simulink model "HybridFEMModel"  (Simulink 7.0)
settings: Solver=FixedStepDiscrete  SolverMode=SingleTasking  StartTime=0.0  StopTime=RunningTime  FixedStep=SampleRate  RelTol=1e-3
values from neighbouring files (symbols this model uses):
  SampleRate = Integrator.Timestep    [HybridFEMSetup_2.m]
undefined symbols (not defined in the file or in its folder): Elements
libraries: simulink x2
(part 1 of 3)
settings Model: Creator=Tommy  LastModifiedBy=Tommy

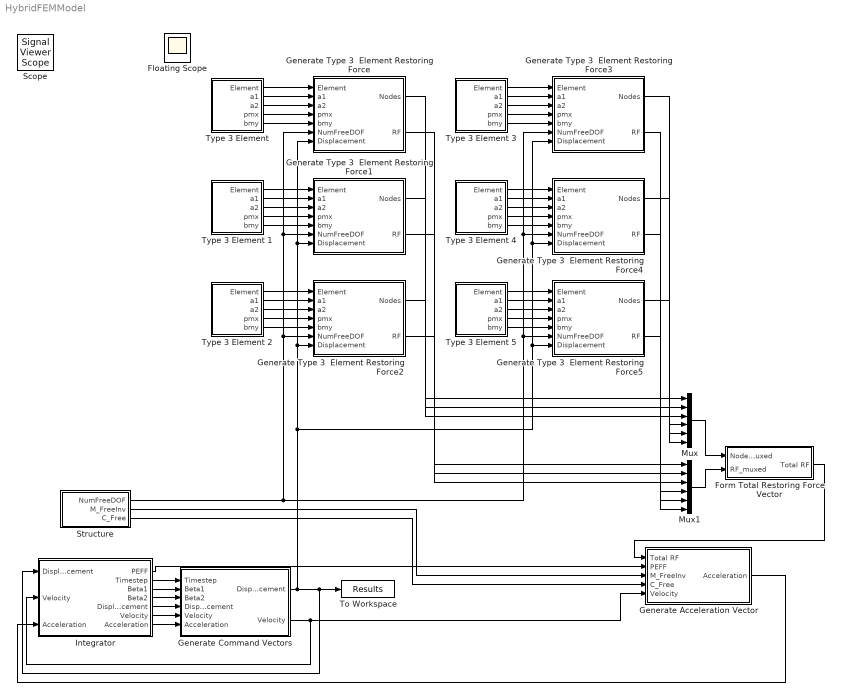
== system HybridFEMModel ==
  Form Total Restoring Force Vector : Subsystem
      mask Type: Form Restoring Force Vector
      mask Description:
      | Takes the restoring force vectors from each Element and combines them to form a total restoring force vector.
      | 
      | Connect the "Nodes_muxed" signal to the output of a Mux block which takes in all the Element "Nodes" outputs in order of ID.
      | 
      | Connect the "RF_muxed" signal to the output of a Mux block which takes in all the Element "RF" outputs in order of ID.
  Generate Acceleration Vector : Subsystem
      mask Type: Generate Acceleration Vector
      mask Description:
      | Takes the total restoring force vector and Integration parameters and generates the next step acceleration vector.
      | 
      | Connect the "Total RF" input to the output of the "Form Total Restoring Force Vector" block.
      | 
      | Connect the "PEFF", "M_Free_Inv" (MassMatrixFreeInv) and "C_Free" (DampingMatrixFree) to the "Structure" block.
      | 
      | Connect the "Velocity" input to the output of the "Generate Command Vectors" block
  Generate Command Vectors : Subsystem
      mask Type: Generate Command Vectors
      mask Description:
      | Generates the Displacement and Velocity vectors using the CR Algorithm.
      | 
      | Connect all inputs to the outputs of the "Integrator" block.
  Generate Type 3  Element Restoring Force : Subsystem
      mask Type: Generate Type 3 Element Restoring Force
      mask Description:
      | Generates the Restoring Force vector for a Type 3 Element
      | 
      | Connect the "Element" input to a "Type 3 Element" block.
      | 
      | Connect the "a1", "a2", "pmx" and "bmy" inputs to the outputs of the "Type 3 Element" block.
      | 
      | Connect the "NumFreeDOF" input to the output of a "Structure" block.
      | 
      | Connect the "Displacement" input to the output of the "Generate Command Vectors" block.
  Generate Type 3  Element Restoring Force1 : Subsystem
      mask Type: Generate Type 3 Element Restoring Force
      mask Description:
      | Generates the Restoring Force vector for a Type 3 Element
      | 
      | Connect the "Element" input to a "Type 3 Element" block.
      | 
      | Connect the "a1", "a2", "pmx" and "bmy" inputs to the outputs of the "Type 3 Element" block.
      | 
      | Connect the "NumFreeDOF" input to the output of a "Structure" block.
      | 
      | Connect the "Displacement" input to the output of the "Generate Command Vectors" block.
  Generate Type 3  Element Restoring Force2 : Subsystem
      mask Type: Generate Type 3 Element Restoring Force
      mask Description:
      | Generates the Restoring Force vector for a Type 3 Element
      | 
      | Connect the "Element" input to a "Type 3 Element" block.
      | 
      | Connect the "a1", "a2", "pmx" and "bmy" inputs to the outputs of the "Type 3 Element" block.
      | 
      | Connect the "NumFreeDOF" input to the output of a "Structure" block.
      | 
      | Connect the "Displacement" input to the output of the "Generate Command Vectors" block.
  Generate Type 3  Element Restoring Force3 : Subsystem
      mask Type: Generate Type 3 Element Restoring Force
      mask Description:
      | Generates the Restoring Force vector for a Type 3 Element
      | 
      | Connect the "Element" input to a "Type 3 Element" block.
      | 
      | Connect the "a1", "a2", "pmx" and "bmy" inputs to the outputs of the "Type 3 Element" block.
      | 
      | Connect the "NumFreeDOF" input to the output of a "Structure" block.
      | 
      | Connect the "Displacement" input to the output of the "Generate Command Vectors" block.
  Generate Type 3  Element Restoring Force4 : Subsystem
      mask Type: Generate Type 3 Element Restoring Force
      mask Description:
      | Generates the Restoring Force vector for a Type 3 Element
      | 
      | Connect the "Element" input to a "Type 3 Element" block.
      | 
      | Connect the "a1", "a2", "pmx" and "bmy" inputs to the outputs of the "Type 3 Element" block.
      | 
      | Connect the "NumFreeDOF" input to the output of a "Structure" block.
      | 
      | Connect the "Displacement" input to the output of the "Generate Command Vectors" block.
  Generate Type 3  Element Restoring Force5 : Subsystem
      mask Type: Generate Type 3 Element Restoring Force
      mask Description:
      | Generates the Restoring Force vector for a Type 3 Element
      | 
      | Connect the "Element" input to a "Type 3 Element" block.
      | 
      | Connect the "a1", "a2", "pmx" and "bmy" inputs to the outputs of the "Type 3 Element" block.
      | 
      | Connect the "NumFreeDOF" input to the output of a "Structure" block.
      | 
      | Connect the "Displacement" input to the output of the "Generate Command Vectors" block.
  Integrator : Subsystem
      mask Type: Integrator
      mask Description:
      | The Integrator structure is pulled from the MATLAB workspace after running the initialization script.
      | 
      | Connect the Displacement and Velocity inputs to the outputs of the "Generate Command Vectors" block.
      | 
      | Connect the Acceleration input to the output of the "Generate Acceleration Vector" block
  Mux : Mux  Inputs=6
  Mux1 : Mux  Inputs=6
  Structure : Subsystem
      mask Type: Structure Data Source
      mask Description: The Structure data is pulled from the MATLAB workspace after running the initialization file
  To Workspace : ToWorkspace  VariableName=Results  SampleTime=SampleRate  SaveFormat=Array
  "Type 3 Element " : Subsystem  mask(Element Type 3){id=1}
      mask prompts: id "Element ID:"
      mask help: Enter the ID for this element corresponding with the input configuration file
  Type 3 Element 1 : Subsystem  mask(Element Type 3){id=2}
      mask prompts: id "Element ID:"
      mask help: Enter the ID for this element corresponding with the input configuration file
  Type 3 Element 2 : Subsystem  mask(Element Type 3){id=3}
      mask prompts: id "Element ID:"
      mask help: Enter the ID for this element corresponding with the input configuration file
  Type 3 Element 3 : Subsystem  mask(Element Type 3){id=4}
      mask prompts: id "Element ID:"
      mask help: Enter the ID for this element corresponding with the input configuration file
  Type 3 Element 4 : Subsystem  mask(Element Type 3){id=5}
      mask prompts: id "Element ID:"
      mask help: Enter the ID for this element corresponding with the input configuration file
  Type 3 Element 5 : Subsystem  mask(Element Type 3){id=6}
      mask prompts: id "Element ID:"
      mask help: Enter the ID for this element corresponding with the input configuration file
  Floating Scope : Scope
      settings: Floating=on
  Scope : SignalViewerScope  IOType=viewer  RefreshTime=0.035000
  wires:
  Integrator/5(Displacement) -> Generate Command Vectors/4("Displacement ")
  Generate Command Vectors/1(Displacement) -> Integrator/1("Displacement "), To Workspace/1, Generate Type 3  Element Restoring Force2/7(Displacement), Generate Type 3  Element Restoring Force1/7(Displacement), Generate Type 3  Element Restoring Force/7(Displacement), Generate Type 3  Element Restoring Force5/7(Displacement), Generate Type 3  Element Restoring Force4/7(Displacement), Generate Type 3  Element Restoring Force3/7(Displacement)
  Form Total Restoring Force Vector/1(Total RF) -> Generate Acceleration Vector/1(Total RF)
  Mux/1 -> Form Total Restoring Force Vector/1(Nodes_Muxed)
  Mux1/1 -> Form Total Restoring Force Vector/2(RF_muxed)
  Integrator/1(PEFF) -> Generate Acceleration Vector/2(PEFF)
  Generate Command Vectors/2(Velocity) -> Integrator/2("Velocity "), Generate Acceleration Vector/5(Velocity)
  Structure/2(M_FreeInv) -> Generate Acceleration Vector/3(M_FreeInv)
  Structure/3(C_Free) -> Generate Acceleration Vector/4(C_Free)
  Generate Acceleration Vector/1(Acceleration) -> Integrator/3("Acceleration ")
  Integrator/2(Timestep) -> Generate Command Vectors/1(Timestep)
  Integrator/3(Beta1) -> Generate Command Vectors/2(Beta1)
  Integrator/4(Beta2) -> Generate Command Vectors/3(Beta2)
  Integrator/6(Velocity) -> Generate Command Vectors/5("Velocity ")
  Integrator/7(Acceleration) -> Generate Command Vectors/6(Acceleration)
  "Type 3 Element "/1(Element) -> Generate Type 3  Element Restoring Force/1(Element)
  "Type 3 Element "/2(a1) -> Generate Type 3  Element Restoring Force/2(a1)
  "Type 3 Element "/3(a2) -> Generate Type 3  Element Restoring Force/3(a2)
  "Type 3 Element "/4(pmx) -> Generate Type 3  Element Restoring Force/4(pmx)
  Type 3 Element 1/1(Element) -> Generate Type 3  Element Restoring Force1/1(Element)
  Type 3 Element 1/2(a1) -> Generate Type 3  Element Restoring Force1/2(a1)
  Type 3 Element 1/3(a2) -> Generate Type 3  Element Restoring Force1/3(a2)
  Type 3 Element 1/4(pmx) -> Generate Type 3  Element Restoring Force1/4(pmx)
  Type 3 Element 1/5(bmy) -> Generate Type 3  Element Restoring Force1/5(bmy)
  Type 3 Element 2/1(Element) -> Generate Type 3  Element Restoring Force2/1(Element)
  Type 3 Element 2/2(a1) -> Generate Type 3  Element Restoring Force2/2(a1)
  Type 3 Element 2/3(a2) -> Generate Type 3  Element Restoring Force2/3(a2)
  Type 3 Element 2/4(pmx) -> Generate Type 3  Element Restoring Force2/4(pmx)
  Type 3 Element 2/5(bmy) -> Generate Type 3  Element Restoring Force2/5(bmy)
  Type 3 Element 3/1(Element) -> Generate Type 3  Element Restoring Force3/1(Element)
  Type 3 Element 3/2(a1) -> Generate Type 3  Element Restoring Force3/2(a1)
  Type 3 Element 3/3(a2) -> Generate Type 3  Element Restoring Force3/3(a2)
  Type 3 Element 3/4(pmx) -> Generate Type 3  Element Restoring Force3/4(pmx)
  Type 3 Element 3/5(bmy) -> Generate Type 3  Element Restoring Force3/5(bmy)
  Type 3 Element 4/1(Element) -> Generate Type 3  Element Restoring Force4/1(Element)
  Type 3 Element 4/2(a1) -> Generate Type 3  Element Restoring Force4/2(a1)
  Type 3 Element 4/3(a2) -> Generate Type 3  Element Restoring Force4/3(a2)
  Type 3 Element 4/4(pmx) -> Generate Type 3  Element Restoring Force4/4(pmx)
  Type 3 Element 4/5(bmy) -> Generate Type 3  Element Restoring Force4/5(bmy)
  Type 3 Element 5/1(Element) -> Generate Type 3  Element Restoring Force5/1(Element)
  Type 3 Element 5/2(a1) -> Generate Type 3  Element Restoring Force5/2(a1)
  Type 3 Element 5/3(a2) -> Generate Type 3  Element Restoring Force5/3(a2)
  Type 3 Element 5/4(pmx) -> Generate Type 3  Element Restoring Force5/4(pmx)
  Type 3 Element 5/5(bmy) -> Generate Type 3  Element Restoring Force5/5(bmy)
  "Type 3 Element "/5(bmy) -> Generate Type 3  Element Restoring Force/5(bmy)
  Structure/1(NumFreeDOF) -> Generate Type 3  Element Restoring Force/6(NumFreeDOF), Generate Type 3  Element Restoring Force1/6(NumFreeDOF), Generate Type 3  Element Restoring Force2/6(NumFreeDOF), Generate Type 3  Element Restoring Force3/6(NumFreeDOF), Generate Type 3  Element Restoring Force4/6(NumFreeDOF), Generate Type 3  Element Restoring Force5/6(NumFreeDOF)
  Generate Type 3  Element Restoring Force/1(Nodes) -> Mux/1
  Generate Type 3  Element Restoring Force1/1(Nodes) -> Mux/2
  Generate Type 3  Element Restoring Force2/1(Nodes) -> Mux/3
  Generate Type 3  Element Restoring Force3/1(Nodes) -> Mux/4
  Generate Type 3  Element Restoring Force4/1(Nodes) -> Mux/5
  Generate Type 3  Element Restoring Force5/1(Nodes) -> Mux/6
  Generate Type 3  Element Restoring Force/2(RF) -> Mux1/1
  Generate Type 3  Element Restoring Force1/2(RF) -> Mux1/2
  Generate Type 3  Element Restoring Force2/2(RF) -> Mux1/3
  Generate Type 3  Element Restoring Force3/2(RF) -> Mux1/4
  Generate Type 3  Element Restoring Force4/2(RF) -> Mux1/5
  Generate Type 3  Element Restoring Force5/2(RF) -> Mux1/6

== system HybridFEMModel/Form Total Restoring Force Vector ==
  Nodes_Muxed : Inport  OutDataType=sfix(16)  OutScaling=2^0
  RF_muxed : Inport  Port=2  OutDataType=sfix(16)  OutScaling=2^0
  Form Restoring Force Vector : Stateflow chart
  Total RF : Outport  OutDataType=sfix(16)  OutScaling=2^0
  wires:
  RF_muxed/1 -> Form Restoring Force Vector/2(RF_muxed)
  Form Restoring Force Vector/1(TotalRF) -> Total RF/1
  Nodes_Muxed/1 -> Form Restoring Force Vector/1(Nodes_muxed)

== system HybridFEMModel/Generate Acceleration Vector ==
  Total RF : Inport  OutDataType=sfix(16)  OutScaling=2^0
  PEFF : Inport  Port=2  OutDataType=sfix(16)  OutScaling=2^0
  M_FreeInv : Inport  Port=3  OutDataType=sfix(16)  OutScaling=2^0
  C_Free : Inport  Port=4  OutDataType=sfix(16)  OutScaling=2^0
  Velocity : Inport  Port=5  OutDataType=sfix(16)  OutScaling=2^0
  Generate Acceleration Vector : Stateflow chart
  Step Count : Subsystem
      mask Type: Step count
      mask Description: Generates the step count
  Acceleration : Outport  OutDataType=sfix(16)  OutScaling=2^0
  wires:
  Step Count/1(Step Count) -> Generate Acceleration Vector/6(step_count)
  Total RF/1 -> Generate Acceleration Vector/1(TotalRF)
  Generate Acceleration Vector/1(Acceleration) -> Acceleration/1
  PEFF/1 -> Generate Acceleration Vector/2(PEFF)
  M_FreeInv/1 -> Generate Acceleration Vector/3(M_FreeInv)
  C_Free/1 -> Generate Acceleration Vector/4(C_Free)
  Velocity/1 -> Generate Acceleration Vector/5(Velocity)

== system HybridFEMModel/Generate Command Vectors ==
  Timestep : Inport  OutDataType=sfix(16)  OutScaling=2^0
  Beta1 : Inport  Port=2  OutDataType=sfix(16)  OutScaling=2^0
  Beta2 : Inport  Port=3  OutDataType=sfix(16)  OutScaling=2^0
  "Displacement " : Inport  Port=4  OutDataType=sfix(16)  OutScaling=2^0
  "Velocity " : Inport  Port=5  OutDataType=sfix(16)  OutScaling=2^0
  Acceleration : Inport  Port=6  OutDataType=sfix(16)  OutScaling=2^0
  Generate Command Vectors : Stateflow chart
  Displacement : Outport  OutDataType=sfix(16)  OutScaling=2^0
  Velocity : Outport  Port=2  OutDataType=sfix(16)  OutScaling=2^0
  wires:
  Generate Command Vectors/1(Displacement_v) -> Displacement/1
  Generate Command Vectors/2(Velocity_v) -> Velocity/1
  Timestep/1 -> Generate Command Vectors/1(Timestep)
  Beta1/1 -> Generate Command Vectors/2(Beta1)
  Beta2/1 -> Generate Command Vectors/3(Beta2)
  "Displacement "/1 -> Generate Command Vectors/4(Displacement)
  "Velocity "/1 -> Generate Command Vectors/5(Velocity)
  Acceleration/1 -> Generate Command Vectors/6(Acceleration)

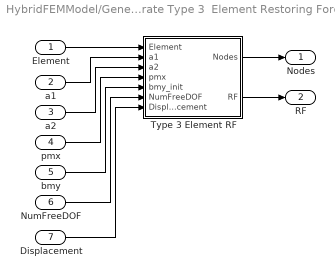
== system HybridFEMModel/Generate Type 3  Element Restoring Force ==
  Element : Inport  OutDataType=sfix(16)  OutScaling=2^0
  a1 : Inport  Port=2  OutDataType=sfix(16)  OutScaling=2^0
  a2 : Inport  Port=3  OutDataType=sfix(16)  OutScaling=2^0
  pmx : Inport  Port=4  OutDataType=sfix(16)  OutScaling=2^0
  bmy : Inport  Port=5  OutDataType=sfix(16)  OutScaling=2^0
  NumFreeDOF : Inport  Port=6  OutDataType=sfix(16)  OutScaling=2^0
  Displacement : Inport  Port=7  OutDataType=sfix(16)  OutScaling=2^0
  Type 3 Element RF : Stateflow chart
  Nodes : Outport  OutDataType=sfix(16)  OutScaling=2^0
  RF : Outport  Port=2  OutDataType=sfix(16)  OutScaling=2^0
  wires:
  Type 3 Element RF/1(Nodes) -> Nodes/1
  Type 3 Element RF/2(RF) -> RF/1
  Element/1 -> Type 3 Element RF/1(Element)
  a1/1 -> Type 3 Element RF/2(a1)
  a2/1 -> Type 3 Element RF/3(a2)
  pmx/1 -> Type 3 Element RF/4(pmx)
  bmy/1 -> Type 3 Element RF/5(bmy_init)
  NumFreeDOF/1 -> Type 3 Element RF/6(NumFreeDOF)
  Displacement/1 -> Type 3 Element RF/7(Displacement)

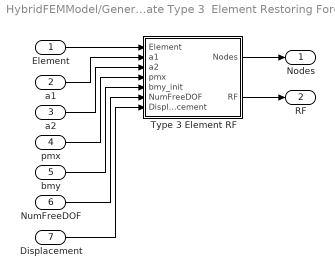
== system HybridFEMModel/Generate Type 3  Element Restoring Force1 ==
  Element : Inport  OutDataType=sfix(16)  OutScaling=2^0
  a1 : Inport  Port=2  OutDataType=sfix(16)  OutScaling=2^0
  a2 : Inport  Port=3  OutDataType=sfix(16)  OutScaling=2^0
  pmx : Inport  Port=4  OutDataType=sfix(16)  OutScaling=2^0
  bmy : Inport  Port=5  OutDataType=sfix(16)  OutScaling=2^0
  NumFreeDOF : Inport  Port=6  OutDataType=sfix(16)  OutScaling=2^0
  Displacement : Inport  Port=7  OutDataType=sfix(16)  OutScaling=2^0
  Type 3 Element RF : Stateflow chart
  Nodes : Outport  OutDataType=sfix(16)  OutScaling=2^0
  RF : Outport  Port=2  OutDataType=sfix(16)  OutScaling=2^0
  wires:
  Displacement/1 -> Type 3 Element RF/7(Displacement)
  NumFreeDOF/1 -> Type 3 Element RF/6(NumFreeDOF)
  bmy/1 -> Type 3 Element RF/5(bmy_init)
  pmx/1 -> Type 3 Element RF/4(pmx)
  a2/1 -> Type 3 Element RF/3(a2)
  a1/1 -> Type 3 Element RF/2(a1)
  Element/1 -> Type 3 Element RF/1(Element)
  Type 3 Element RF/2(RF) -> RF/1
  Type 3 Element RF/1(Nodes) -> Nodes/1

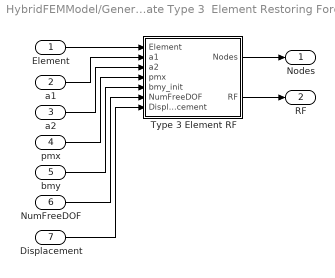
== system HybridFEMModel/Generate Type 3  Element Restoring Force2 ==
  Element : Inport  OutDataType=sfix(16)  OutScaling=2^0
  a1 : Inport  Port=2  OutDataType=sfix(16)  OutScaling=2^0
  a2 : Inport  Port=3  OutDataType=sfix(16)  OutScaling=2^0
  pmx : Inport  Port=4  OutDataType=sfix(16)  OutScaling=2^0
  bmy : Inport  Port=5  OutDataType=sfix(16)  OutScaling=2^0
  NumFreeDOF : Inport  Port=6  OutDataType=sfix(16)  OutScaling=2^0
  Displacement : Inport  Port=7  OutDataType=sfix(16)  OutScaling=2^0
  Type 3 Element RF : Stateflow chart
  Nodes : Outport  OutDataType=sfix(16)  OutScaling=2^0
  RF : Outport  Port=2  OutDataType=sfix(16)  OutScaling=2^0
  wires:
  Type 3 Element RF/1(Nodes) -> Nodes/1
  Type 3 Element RF/2(RF) -> RF/1
  Element/1 -> Type 3 Element RF/1(Element)
  a1/1 -> Type 3 Element RF/2(a1)
  a2/1 -> Type 3 Element RF/3(a2)
  pmx/1 -> Type 3 Element RF/4(pmx)
  bmy/1 -> Type 3 Element RF/5(bmy_init)
  NumFreeDOF/1 -> Type 3 Element RF/6(NumFreeDOF)
  Displacement/1 -> Type 3 Element RF/7(Displacement)

== system HybridFEMModel/Generate Type 3  Element Restoring Force3 ==
  Element : Inport  OutDataType=sfix(16)  OutScaling=2^0
  a1 : Inport  Port=2  OutDataType=sfix(16)  OutScaling=2^0
  a2 : Inport  Port=3  OutDataType=sfix(16)  OutScaling=2^0
  pmx : Inport  Port=4  OutDataType=sfix(16)  OutScaling=2^0
  bmy : Inport  Port=5  OutDataType=sfix(16)  OutScaling=2^0
  NumFreeDOF : Inport  Port=6  OutDataType=sfix(16)  OutScaling=2^0
  Displacement : Inport  Port=7  OutDataType=sfix(16)  OutScaling=2^0
  Type 3 Element RF : Stateflow chart
  Nodes : Outport  OutDataType=sfix(16)  OutScaling=2^0
  RF : Outport  Port=2  OutDataType=sfix(16)  OutScaling=2^0
  wires:
  Displacement/1 -> Type 3 Element RF/7(Displacement)
  NumFreeDOF/1 -> Type 3 Element RF/6(NumFreeDOF)
  bmy/1 -> Type 3 Element RF/5(bmy_init)
  pmx/1 -> Type 3 Element RF/4(pmx)
  a2/1 -> Type 3 Element RF/3(a2)
  a1/1 -> Type 3 Element RF/2(a1)
  Element/1 -> Type 3 Element RF/1(Element)
  Type 3 Element RF/2(RF) -> RF/1
  Type 3 Element RF/1(Nodes) -> Nodes/1

== system HybridFEMModel/Generate Type 3  Element Restoring Force4 ==
  Element : Inport  OutDataType=sfix(16)  OutScaling=2^0
  a1 : Inport  Port=2  OutDataType=sfix(16)  OutScaling=2^0
  a2 : Inport  Port=3  OutDataType=sfix(16)  OutScaling=2^0
  pmx : Inport  Port=4  OutDataType=sfix(16)  OutScaling=2^0
  bmy : Inport  Port=5  OutDataType=sfix(16)  OutScaling=2^0
  NumFreeDOF : Inport  Port=6  OutDataType=sfix(16)  OutScaling=2^0
  Displacement : Inport  Port=7  OutDataType=sfix(16)  OutScaling=2^0
  Type 3 Element RF : Stateflow chart
  Nodes : Outport  OutDataType=sfix(16)  OutScaling=2^0
  RF : Outport  Port=2  OutDataType=sfix(16)  OutScaling=2^0
  wires:
  Type 3 Element RF/1(Nodes) -> Nodes/1
  Type 3 Element RF/2(RF) -> RF/1
  Element/1 -> Type 3 Element RF/1(Element)
  a1/1 -> Type 3 Element RF/2(a1)
  a2/1 -> Type 3 Element RF/3(a2)
  pmx/1 -> Type 3 Element RF/4(pmx)
  bmy/1 -> Type 3 Element RF/5(bmy_init)
  NumFreeDOF/1 -> Type 3 Element RF/6(NumFreeDOF)
  Displacement/1 -> Type 3 Element RF/7(Displacement)

== system HybridFEMModel/Generate Type 3  Element Restoring Force5 ==
  Element : Inport  OutDataType=sfix(16)  OutScaling=2^0
  a1 : Inport  Port=2  OutDataType=sfix(16)  OutScaling=2^0
  a2 : Inport  Port=3  OutDataType=sfix(16)  OutScaling=2^0
  pmx : Inport  Port=4  OutDataType=sfix(16)  OutScaling=2^0
  bmy : Inport  Port=5  OutDataType=sfix(16)  OutScaling=2^0
  NumFreeDOF : Inport  Port=6  OutDataType=sfix(16)  OutScaling=2^0
  Displacement : Inport  Port=7  OutDataType=sfix(16)  OutScaling=2^0
  Type 3 Element RF : Stateflow chart
  Nodes : Outport  OutDataType=sfix(16)  OutScaling=2^0
  RF : Outport  Port=2  OutDataType=sfix(16)  OutScaling=2^0
  wires:
  Displacement/1 -> Type 3 Element RF/7(Displacement)
  NumFreeDOF/1 -> Type 3 Element RF/6(NumFreeDOF)
  bmy/1 -> Type 3 Element RF/5(bmy_init)
  pmx/1 -> Type 3 Element RF/4(pmx)
  a2/1 -> Type 3 Element RF/3(a2)
  a1/1 -> Type 3 Element RF/2(a1)
  Element/1 -> Type 3 Element RF/1(Element)
  Type 3 Element RF/2(RF) -> RF/1
  Type 3 Element RF/1(Nodes) -> Nodes/1

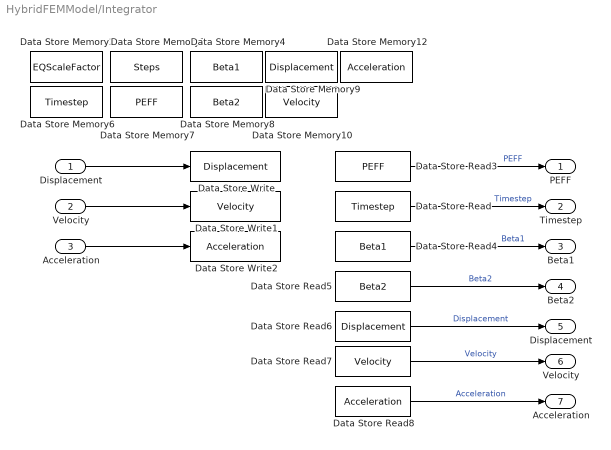
== system HybridFEMModel/Integrator ==
  "Displacement " : Inport  OutDataType=sfix(16)  OutScaling=2^0
  "Velocity " : Inport  Port=2  OutDataType=sfix(16)  OutScaling=2^0
  "Acceleration " : Inport  Port=3  OutDataType=sfix(16)  OutScaling=2^0
  Data Store Memory10 : DataStoreMemory  DataStoreName=Velocity  InitialValue=Integrator.Velocity  OutDataType=sfix(16)  OutScaling=2^0
  Data Store Memory12 : DataStoreMemory  DataStoreName=Acceleration  InitialValue=Integrator.Acceleration  OutDataType=sfix(16)  OutScaling=2^0
  Data Store Memory2 : DataStoreMemory  DataStoreName=EQScaleFactor  InitialValue=Integrator.EQScaleFactor  OutDataType=sfix(16)  OutScaling=2^0
  Data Store Memory3 : DataStoreMemory  DataStoreName=Steps  InitialValue=Integrator.Steps  OutDataType=sfix(16)  OutScaling=2^0
  Data Store Memory4 : DataStoreMemory  DataStoreName=Beta1  InitialValue=Integrator.Beta1  OutDataType=sfix(16)  OutScaling=2^0
  Data Store Memory6 : DataStoreMemory  DataStoreName=Timestep  InitialValue=Integrator.Timestep  OutDataType=sfix(16)  OutScaling=2^0
  Data Store Memory7 : DataStoreMemory  DataStoreName=PEFF  InitialValue=Integrator.PEFF  OutDataType=sfix(16)  OutScaling=2^0
  Data Store Memory8 : DataStoreMemory  DataStoreName=Beta2  InitialValue=Integrator.Beta2  OutDataType=sfix(16)  OutScaling=2^0
  Data Store Memory9 : DataStoreMemory  DataStoreName=Displacement  InitialValue=Integrator.Displacement  OutDataType=sfix(16)  OutScaling=2^0
  Data Store Read : DataStoreRead  DataStoreName=Timestep  SampleTime=SampleRate
  Data Store Read3 : DataStoreRead  DataStoreName=PEFF  SampleTime=SampleRate
  Data Store Read4 : DataStoreRead  DataStoreName=Beta1  SampleTime=SampleRate
  Data Store Read5 : DataStoreRead  DataStoreName=Beta2  SampleTime=SampleRate
  Data Store Read6 : DataStoreRead  DataStoreName=Displacement  SampleTime=SampleRate
  Data Store Read7 : DataStoreRead  DataStoreName=Velocity  SampleTime=SampleRate
  Data Store Read8 : DataStoreRead  DataStoreName=Acceleration  SampleTime=SampleRate
  Data Store Write : DataStoreWrite  DataStoreName=Displacement  SampleTime=SampleRate
  Data Store Write1 : DataStoreWrite  DataStoreName=Velocity  SampleTime=SampleRate
  Data Store Write2 : DataStoreWrite  DataStoreName=Acceleration  SampleTime=SampleRate
  PEFF : Outport  OutDataType=sfix(16)  OutScaling=2^0
  Timestep : Outport  Port=2  OutDataType=sfix(16)  OutScaling=2^0
  Beta1 : Outport  Port=3  OutDataType=sfix(16)  OutScaling=2^0
  Beta2 : Outport  Port=4  OutDataType=sfix(16)  OutScaling=2^0
  Displacement : Outport  Port=5  OutDataType=sfix(16)  OutScaling=2^0
  Velocity : Outport  Port=6  OutDataType=sfix(16)  OutScaling=2^0
  Acceleration : Outport  Port=7  OutDataType=sfix(16)  OutScaling=2^0
  wires:
  Data Store Read/1 -> Timestep/1  "Timestep"
  "Acceleration "/1 -> Data Store Write2/1
  "Velocity "/1 -> Data Store Write1/1
  "Displacement "/1 -> Data Store Write/1
  Data Store Read3/1 -> PEFF/1  "PEFF"
  Data Store Read4/1 -> Beta1/1  "Beta1"
  Data Store Read5/1 -> Beta2/1  "Beta2"
  Data Store Read6/1 -> Displacement/1  "Displacement"
  Data Store Read7/1 -> Velocity/1  "Velocity"
  Data Store Read8/1 -> Acceleration/1  "Acceleration"

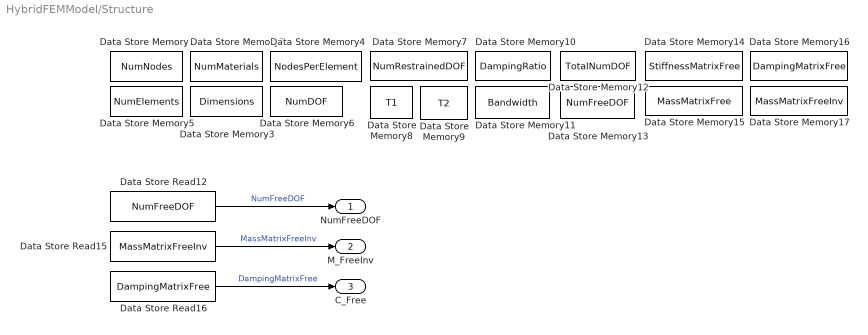
== system HybridFEMModel/Structure ==
  Data Store Memory1 : DataStoreMemory  DataStoreName=NumNodes  InitialValue=Structure.NumNodes  OutDataType=sfix(16)  OutScaling=2^0
  Data Store Memory10 : DataStoreMemory  DataStoreName=DampingRatio  InitialValue=Structure.DampingRatio  OutDataType=sfix(16)  OutScaling=2^0
  Data Store Memory11 : DataStoreMemory  DataStoreName=Bandwidth  InitialValue=Structure.Bandwidth  OutDataType=sfix(16)  OutScaling=2^0
  Data Store Memory12 : DataStoreMemory  DataStoreName=TotalNumDOF  InitialValue=Structure.TotalNumDOF  OutDataType=sfix(16)  OutScaling=2^0
  Data Store Memory13 : DataStoreMemory  DataStoreName=NumFreeDOF  InitialValue=Structure.NumFreeDOF  OutDataType=sfix(16)  OutScaling=2^0
  Data Store Memory14 : DataStoreMemory  DataStoreName=StiffnessMatrixFree  InitialValue=Structure.StiffnessMatrixFree  OutDataType=sfix(16)  OutScaling=2^0
  Data Store Memory15 : DataStoreMemory  DataStoreName=MassMatrixFree  InitialValue=Structure.MassMatrixFree  OutDataType=sfix(16)  OutScaling=2^0
  Data Store Memory16 : DataStoreMemory  DataStoreName=DampingMatrixFree  InitialValue=Structure.DampingMatrixFree  OutDataType=sfix(16)  OutScaling=2^0
  Data Store Memory17 : DataStoreMemory  DataStoreName=MassMatrixFreeInv  InitialValue=Structure.MassMatrixFreeInv  OutDataType=sfix(16)  OutScaling=2^0
  Data Store Memory2 : DataStoreMemory  DataStoreName=NumMaterials  InitialValue=Structure.NumMaterials  OutDataType=sfix(16)  OutScaling=2^0
  Data Store Memory3 : DataStoreMemory  DataStoreName=Dimensions  InitialValue=Structure.Dimensions  OutDataType=sfix(16)  OutScaling=2^0
  Data Store Memory4 : DataStoreMemory  DataStoreName=NodesPerElement  InitialValue=Structure.NodesPerElement  OutDataType=sfix(16)  OutScaling=2^0
  Data Store Memory5 : DataStoreMemory  DataStoreName=NumElements  InitialValue=Structure.NumElements  OutDataType=sfix(16)  OutScaling=2^0
  Data Store Memory6 : DataStoreMemory  DataStoreName=NumDOF  InitialValue=Structure.NumDOF  OutDataType=sfix(16)  OutScaling=2^0
  Data Store Memory7 : DataStoreMemory  DataStoreName=NumRestrainedDOF  InitialValue=Structure.NumRestrainedDOF  OutDataType=sfix(16)  OutScaling=2^0
  Data Store Memory8 : DataStoreMemory  DataStoreName=T1  InitialValue=Structure.T1  OutDataType=sfix(16)  OutScaling=2^0
  Data Store Memory9 : DataStoreMemory  DataStoreName=T2  InitialValue=Structure.T2  OutDataType=sfix(16)  OutScaling=2^0
  Data Store Read12 : DataStoreRead  DataStoreName=NumFreeDOF  SampleTime=SampleRate
  Data Store Read15 : DataStoreRead  DataStoreName=MassMatrixFreeInv  SampleTime=SampleRate
  Data Store Read16 : DataStoreRead  DataStoreName=DampingMatrixFree  SampleTime=SampleRate
  NumFreeDOF : Outport  OutDataType=sfix(16)  OutScaling=2^0
  M_FreeInv : Outport  Port=2  OutDataType=sfix(16)  OutScaling=2^0
  C_Free : Outport  Port=3  OutDataType=sfix(16)  OutScaling=2^0
  wires:
  Data Store Read12/1 -> NumFreeDOF/1  "NumFreeDOF"
  Data Store Read15/1 -> M_FreeInv/1  "MassMatrixFreeInv"
  Data Store Read16/1 -> C_Free/1  "DampingMatrixFree"

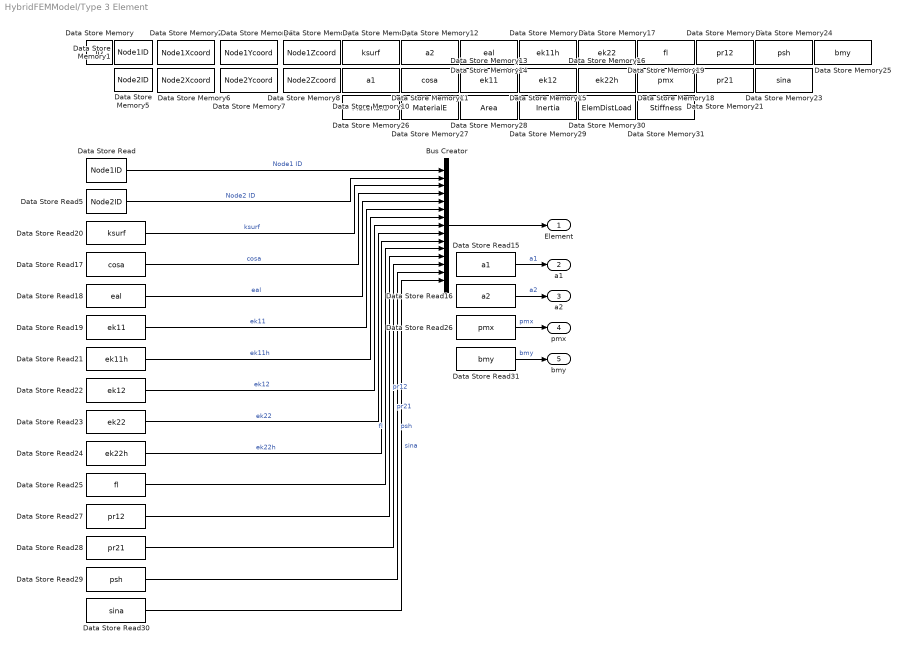
== system HybridFEMModel/Type 3 Element  ==
  Bus Creator : BusCreator  Inputs=15
  Data Store Memory : DataStoreMemory  DataStoreName=ID  InitialValue=Elements(id).ID  OutDataType=sfix(16)  OutScaling=2^0
  Data Store Memory1 : DataStoreMemory  DataStoreName=Node1ID  InitialValue=Elements(id).Nodes(1).ID  OutDataType=sfix(16)  OutScaling=2^0
  Data Store Memory10 : DataStoreMemory  DataStoreName=a1  InitialValue=Elements(id).a1  OutDataType=sfix(16)  OutScaling=2^0
  Data Store Memory11 : DataStoreMemory  DataStoreName=cosa  InitialValue=Elements(id).cosa  OutDataType=sfix(16)  OutScaling=2^0
  Data Store Memory12 : DataStoreMemory  DataStoreName=a2  InitialValue=Elements(id).a2  OutDataType=sfix(16)  OutScaling=2^0
  Data Store Memory13 : DataStoreMemory  DataStoreName=ek11  InitialValue=Elements(id).ek11  OutDataType=sfix(16)  OutScaling=2^0
  Data Store Memory14 : DataStoreMemory  DataStoreName=eal  InitialValue=Elements(id).eal  OutDataType=sfix(16)  OutScaling=2^0
  Data Store Memory15 : DataStoreMemory  DataStoreName=ek12  InitialValue=Elements(id).ek12  OutDataType=sfix(16)  OutScaling=2^0
  Data Store Memory16 : DataStoreMemory  DataStoreName=ek22h  InitialValue=Elements(id).ek22h  OutDataType=sfix(16)  OutScaling=2^0
  Data Store Memory17 : DataStoreMemory  DataStoreName=ek22  InitialValue=Elements(id).ek22  OutDataType=sfix(16)  OutScaling=2^0
  Data Store Memory18 : DataStoreMemory  DataStoreName=pmx  InitialValue=Elements(id).pmx  OutDataType=sfix(16)  OutScaling=2^0
  Data Store Memory19 : DataStoreMemory  DataStoreName=fl  InitialValue=Elements(id).fl  OutDataType=sfix(16)  OutScaling=2^0
  Data Store Memory2 : DataStoreMemory  DataStoreName=Node1Xcoord  InitialValue=Elements(id).Nodes(1).Xcoord  OutDataType=sfix(16)  OutScaling=2^0
  Data Store Memory20 : DataStoreMemory  DataStoreName=ek11h  InitialValue=Elements(id).ek11h  OutDataType=sfix(16)  OutScaling=2^0
  Data Store Memory21 : DataStoreMemory  DataStoreName=pr21  InitialValue=Elements(id).pr21  OutDataType=sfix(16)  OutScaling=2^0
  Data Store Memory22 : DataStoreMemory  DataStoreName=pr12  InitialValue=Elements(id).pr12  OutDataType=sfix(16)  OutScaling=2^0
  Data Store Memory23 : DataStoreMemory  DataStoreName=sina  InitialValue=Elements(id).sina  OutDataType=sfix(16)  OutScaling=2^0
  Data Store Memory24 : DataStoreMemory  DataStoreName=psh  InitialValue=Elements(id).psh  OutDataType=sfix(16)  OutScaling=2^0
  Data Store Memory25 : DataStoreMemory  DataStoreName=bmy  InitialValue=Elements(id).bmy  OutDataType=sfix(16)  OutScaling=2^0
  Data Store Memory26 : DataStoreMemory  DataStoreName=MaterialID  InitialValue=Elements(id).Material.ID  OutDataType=sfix(16)  OutScaling=2^0
  Data Store Memory27 : DataStoreMemory  DataStoreName=MaterialE  InitialValue=Elements(id).Material.E  OutDataType=sfix(16)  OutScaling=2^0
  Data Store Memory28 : DataStoreMemory  DataStoreName=Area  InitialValue=Elements(id).Area  OutDataType=sfix(16)  OutScaling=2^0
  Data Store Memory29 : DataStoreMemory  DataStoreName=Inertia  InitialValue=Elements(id).Inertia  OutDataType=sfix(16)  OutScaling=2^0
  Data Store Memory3 : DataStoreMemory  DataStoreName=Node1Ycoord  InitialValue=Elements(id).Nodes(1).Ycoord  OutDataType=sfix(16)  OutScaling=2^0
  Data Store Memory30 : DataStoreMemory  DataStoreName=ElemDistLoad  InitialValue=Elements(id).ElemDistLoad  OutDataType=sfix(16)  OutScaling=2^0
  Data Store Memory31 : DataStoreMemory  DataStoreName=Stiffness  InitialValue=Elements(id).Stiffness  OutDataType=sfix(16)  OutScaling=2^0
  Data Store Memory4 : DataStoreMemory  DataStoreName=Node1Zcoord  InitialValue=Elements(id).Nodes(1).Zcoord  OutDataType=sfix(16)  OutScaling=2^0
  Data Store Memory5 : DataStoreMemory  DataStoreName=Node2ID  InitialValue=Elements(id).Nodes(2).ID  OutDataType=sfix(16)  OutScaling=2^0
  Data Store Memory6 : DataStoreMemory  DataStoreName=Node2Xcoord  InitialValue=Elements(id).Nodes(2).Xcoord  OutDataType=sfix(16)  OutScaling=2^0
  Data Store Memory7 : DataStoreMemory  DataStoreName=Node2Ycoord  InitialValue=Elements(id).Nodes(2).Ycoord  OutDataType=sfix(16)  OutScaling=2^0
  Data Store Memory8 : DataStoreMemory  DataStoreName=Node2Zcoord  InitialValue=Elements(id).Nodes(2).Zcoord  OutDataType=sfix(16)  OutScaling=2^0
  Data Store Memory9 : DataStoreMemory  DataStoreName=ksurf  InitialValue=Elements(id).ksurf  OutDataType=sfix(16)  OutScaling=2^0
  Data Store Read : DataStoreRead  DataStoreName=Node1ID  SampleTime=SampleRate
  Data Store Read15 : DataStoreRead  DataStoreName=a1  SampleTime=SampleRate
  Data Store Read16 : DataStoreRead  DataStoreName=a2  SampleTime=SampleRate
  Data Store Read17 : DataStoreRead  DataStoreName=cosa  SampleTime=SampleRate
  Data Store Read18 : DataStoreRead  DataStoreName=eal  SampleTime=SampleRate
  Data Store Read19 : DataStoreRead  DataStoreName=ek11  SampleTime=SampleRate
  Data Store Read20 : DataStoreRead  DataStoreName=ksurf  SampleTime=SampleRate
  Data Store Read21 : DataStoreRead  DataStoreName=ek11h  SampleTime=SampleRate
  Data Store Read22 : DataStoreRead  DataStoreName=ek12  SampleTime=SampleRate
  Data Store Read23 : DataStoreRead  DataStoreName=ek22  SampleTime=SampleRate
  Data Store Read24 : DataStoreRead  DataStoreName=ek22h  SampleTime=SampleRate
  Data Store Read25 : DataStoreRead  DataStoreName=fl  SampleTime=SampleRate
  Data Store Read26 : DataStoreRead  DataStoreName=pmx  SampleTime=SampleRate
  Data Store Read27 : DataStoreRead  DataStoreName=pr12  SampleTime=SampleRate
  Data Store Read28 : DataStoreRead  DataStoreName=pr21  SampleTime=SampleRate
  Data Store Read29 : DataStoreRead  DataStoreName=psh  SampleTime=SampleRate
  Data Store Read30 : DataStoreRead  DataStoreName=sina  SampleTime=SampleRate
  Data Store Read31 : DataStoreRead  DataStoreName=bmy  SampleTime=SampleRate
  Data Store Read5 : DataStoreRead  DataStoreName=Node2ID  SampleTime=SampleRate
  Element : Outport  OutDataType=sfix(16)  OutScaling=2^0
  a1 : Outport  Port=2  OutDataType=sfix(16)  OutScaling=2^0
  a2 : Outport  Port=3  OutDataType=sfix(16)  OutScaling=2^0
  pmx : Outport  Port=4  OutDataType=sfix(16)  OutScaling=2^0
  bmy : Outport  Port=5  OutDataType=sfix(16)  OutScaling=2^0
  wires:
  Bus Creator/1 -> Element/1
  Data Store Read/1 -> Bus Creator/1  "Node1 ID"
  Data Store Read5/1 -> Bus Creator/2  "Node2 ID"
  Data Store Read20/1 -> Bus Creator/3  "ksurf"
  Data Store Read17/1 -> Bus Creator/4  "cosa"
  Data Store Read18/1 -> Bus Creator/5  "eal"
  Data Store Read19/1 -> Bus Creator/6  "ek11"
  Data Store Read21/1 -> Bus Creator/7  "ek11h"
  Data Store Read22/1 -> Bus Creator/8  "ek12"
  Data Store Read23/1 -> Bus Creator/9  "ek22"
  Data Store Read24/1 -> Bus Creator/10  "ek22h"
  Data Store Read25/1 -> Bus Creator/11  "fl"
  Data Store Read27/1 -> Bus Creator/12  "pr12"
  Data Store Read28/1 -> Bus Creator/13  "pr21"
  Data Store Read29/1 -> Bus Creator/14  "psh"
  Data Store Read30/1 -> Bus Creator/15  "sina"
  Data Store Read15/1 -> a1/1  "a1"
  Data Store Read16/1 -> a2/1  "a2"
  Data Store Read26/1 -> pmx/1  "pmx"
  Data Store Read31/1 -> bmy/1  "bmy"

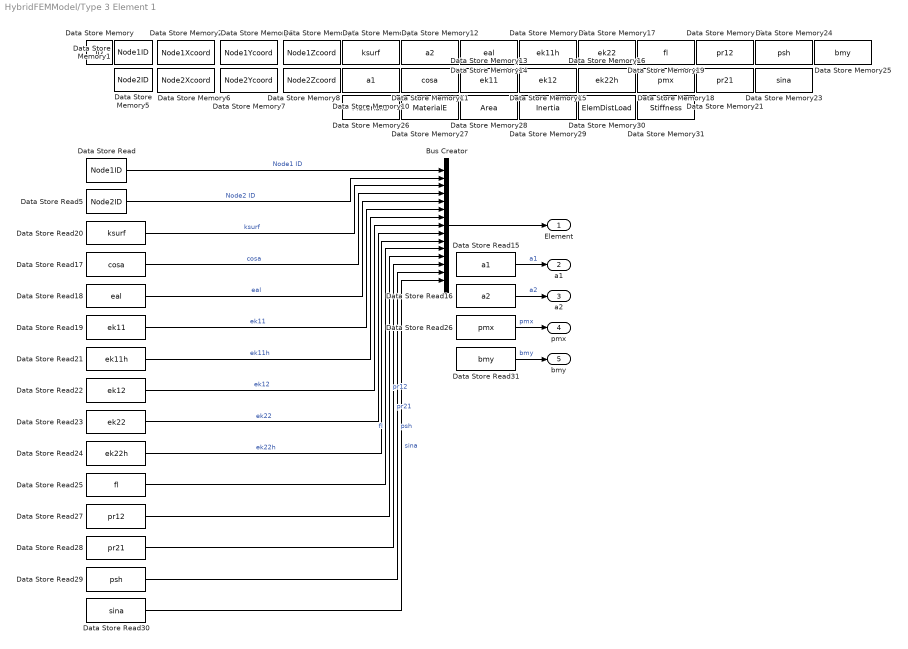
== system HybridFEMModel/Type 3 Element 1 ==
  Bus Creator : BusCreator  Inputs=15
  Data Store Memory : DataStoreMemory  DataStoreName=ID  InitialValue=Elements(id).ID  OutDataType=sfix(16)  OutScaling=2^0
  Data Store Memory1 : DataStoreMemory  DataStoreName=Node1ID  InitialValue=Elements(id).Nodes(1).ID  OutDataType=sfix(16)  OutScaling=2^0
  Data Store Memory10 : DataStoreMemory  DataStoreName=a1  InitialValue=Elements(id).a1  OutDataType=sfix(16)  OutScaling=2^0
  Data Store Memory11 : DataStoreMemory  DataStoreName=cosa  InitialValue=Elements(id).cosa  OutDataType=sfix(16)  OutScaling=2^0
  Data Store Memory12 : DataStoreMemory  DataStoreName=a2  InitialValue=Elements(id).a2  OutDataType=sfix(16)  OutScaling=2^0
  Data Store Memory13 : DataStoreMemory  DataStoreName=ek11  InitialValue=Elements(id).ek11  OutDataType=sfix(16)  OutScaling=2^0
  Data Store Memory14 : DataStoreMemory  DataStoreName=eal  InitialValue=Elements(id).eal  OutDataType=sfix(16)  OutScaling=2^0
  Data Store Memory15 : DataStoreMemory  DataStoreName=ek12  InitialValue=Elements(id).ek12  OutDataType=sfix(16)  OutScaling=2^0
  Data Store Memory16 : DataStoreMemory  DataStoreName=ek22h  InitialValue=Elements(id).ek22h  OutDataType=sfix(16)  OutScaling=2^0
  Data Store Memory17 : DataStoreMemory  DataStoreName=ek22  InitialValue=Elements(id).ek22  OutDataType=sfix(16)  OutScaling=2^0
  Data Store Memory18 : DataStoreMemory  DataStoreName=pmx  InitialValue=Elements(id).pmx  OutDataType=sfix(16)  OutScaling=2^0
  Data Store Memory19 : DataStoreMemory  DataStoreName=fl  InitialValue=Elements(id).fl  OutDataType=sfix(16)  OutScaling=2^0
  Data Store Memory2 : DataStoreMemory  DataStoreName=Node1Xcoord  InitialValue=Elements(id).Nodes(1).Xcoord  OutDataType=sfix(16)  OutScaling=2^0
  Data Store Memory20 : DataStoreMemory  DataStoreName=ek11h  InitialValue=Elements(id).ek11h  OutDataType=sfix(16)  OutScaling=2^0
  Data Store Memory21 : DataStoreMemory  DataStoreName=pr21  InitialValue=Elements(id).pr21  OutDataType=sfix(16)  OutScaling=2^0
  Data Store Memory22 : DataStoreMemory  DataStoreName=pr12  InitialValue=Elements(id).pr12  OutDataType=sfix(16)  OutScaling=2^0
  Data Store Memory23 : DataStoreMemory  DataStoreName=sina  InitialValue=Elements(id).sina  OutDataType=sfix(16)  OutScaling=2^0
  Data Store Memory24 : DataStoreMemory  DataStoreName=psh  InitialValue=Elements(id).psh  OutDataType=sfix(16)  OutScaling=2^0
  Data Store Memory25 : DataStoreMemory  DataStoreName=bmy  InitialValue=Elements(id).bmy  OutDataType=sfix(16)  OutScaling=2^0
  Data Store Memory26 : DataStoreMemory  DataStoreName=MaterialID  InitialValue=Elements(id).Material.ID  OutDataType=sfix(16)  OutScaling=2^0
  Data Store Memory27 : DataStoreMemory  DataStoreName=MaterialE  InitialValue=Elements(id).Material.E  OutDataType=sfix(16)  OutScaling=2^0
  Data Store Memory28 : DataStoreMemory  DataStoreName=Area  InitialValue=Elements(id).Area  OutDataType=sfix(16)  OutScaling=2^0
  Data Store Memory29 : DataStoreMemory  DataStoreName=Inertia  InitialValue=Elements(id).Inertia  OutDataType=sfix(16)  OutScaling=2^0
  Data Store Memory3 : DataStoreMemory  DataStoreName=Node1Ycoord  InitialValue=Elements(id).Nodes(1).Ycoord  OutDataType=sfix(16)  OutScaling=2^0
  Data Store Memory30 : DataStoreMemory  DataStoreName=ElemDistLoad  InitialValue=Elements(id).ElemDistLoad  OutDataType=sfix(16)  OutScaling=2^0
  Data Store Memory31 : DataStoreMemory  DataStoreName=Stiffness  InitialValue=Elements(id).Stiffness  OutDataType=sfix(16)  OutScaling=2^0
  Data Store Memory4 : DataStoreMemory  DataStoreName=Node1Zcoord  InitialValue=Elements(id).Nodes(1).Zcoord  OutDataType=sfix(16)  OutScaling=2^0
  Data Store Memory5 : DataStoreMemory  DataStoreName=Node2ID  InitialValue=Elements(id).Nodes(2).ID  OutDataType=sfix(16)  OutScaling=2^0
  Data Store Memory6 : DataStoreMemory  DataStoreName=Node2Xcoord  InitialValue=Elements(id).Nodes(2).Xcoord  OutDataType=sfix(16)  OutScaling=2^0
  Data Store Memory7 : DataStoreMemory  DataStoreName=Node2Ycoord  InitialValue=Elements(id).Nodes(2).Ycoord  OutDataType=sfix(16)  OutScaling=2^0
  Data Store Memory8 : DataStoreMemory  DataStoreName=Node2Zcoord  InitialValue=Elements(id).Nodes(2).Zcoord  OutDataType=sfix(16)  OutScaling=2^0
  Data Store Memory9 : DataStoreMemory  DataStoreName=ksurf  InitialValue=Elements(id).ksurf  OutDataType=sfix(16)  OutScaling=2^0
  Data Store Read : DataStoreRead  DataStoreName=Node1ID  SampleTime=SampleRate
  Data Store Read15 : DataStoreRead  DataStoreName=a1  SampleTime=SampleRate
  Data Store Read16 : DataStoreRead  DataStoreName=a2  SampleTime=SampleRate
  Data Store Read17 : DataStoreRead  DataStoreName=cosa  SampleTime=SampleRate
  Data Store Read18 : DataStoreRead  DataStoreName=eal  SampleTime=SampleRate
  Data Store Read19 : DataStoreRead  DataStoreName=ek11  SampleTime=SampleRate
  Data Store Read20 : DataStoreRead  DataStoreName=ksurf  SampleTime=SampleRate
  Data Store Read21 : DataStoreRead  DataStoreName=ek11h  SampleTime=SampleRate
  Data Store Read22 : DataStoreRead  DataStoreName=ek12  SampleTime=SampleRate
  Data Store Read23 : DataStoreRead  DataStoreName=ek22  SampleTime=SampleRate
  Data Store Read24 : DataStoreRead  DataStoreName=ek22h  SampleTime=SampleRate
  Data Store Read25 : DataStoreRead  DataStoreName=fl  SampleTime=SampleRate
  Data Store Read26 : DataStoreRead  DataStoreName=pmx  SampleTime=SampleRate
  Data Store Read27 : DataStoreRead  DataStoreName=pr12  SampleTime=SampleRate
  Data Store Read28 : DataStoreRead  DataStoreName=pr21  SampleTime=SampleRate
  Data Store Read29 : DataStoreRead  DataStoreName=psh  SampleTime=SampleRate
  Data Store Read30 : DataStoreRead  DataStoreName=sina  SampleTime=SampleRate
  Data Store Read31 : DataStoreRead  DataStoreName=bmy  SampleTime=SampleRate
  Data Store Read5 : DataStoreRead  DataStoreName=Node2ID  SampleTime=SampleRate
  Element : Outport  OutDataType=sfix(16)  OutScaling=2^0
  a1 : Outport  Port=2  OutDataType=sfix(16)  OutScaling=2^0
  a2 : Outport  Port=3  OutDataType=sfix(16)  OutScaling=2^0
  pmx : Outport  Port=4  OutDataType=sfix(16)  OutScaling=2^0
  bmy : Outport  Port=5  OutDataType=sfix(16)  OutScaling=2^0
  wires:
  Data Store Read31/1 -> bmy/1  "bmy"
  Data Store Read26/1 -> pmx/1  "pmx"
  Data Store Read16/1 -> a2/1  "a2"
  Data Store Read15/1 -> a1/1  "a1"
  Data Store Read30/1 -> Bus Creator/15  "sina"
  Data Store Read29/1 -> Bus Creator/14  "psh"
  Data Store Read28/1 -> Bus Creator/13  "pr21"
  Data Store Read27/1 -> Bus Creator/12  "pr12"
  Data Store Read25/1 -> Bus Creator/11  "fl"
  Data Store Read24/1 -> Bus Creator/10  "ek22h"
  Data Store Read23/1 -> Bus Creator/9  "ek22"
  Data Store Read22/1 -> Bus Creator/8  "ek12"
  Data Store Read21/1 -> Bus Creator/7  "ek11h"
  Data Store Read19/1 -> Bus Creator/6  "ek11"
  Data Store Read18/1 -> Bus Creator/5  "eal"
  Data Store Read17/1 -> Bus Creator/4  "cosa"
  Data Store Read20/1 -> Bus Creator/3  "ksurf"
  Data Store Read5/1 -> Bus Creator/2  "Node2 ID"
  Data Store Read/1 -> Bus Creator/1  "Node1 ID"
  Bus Creator/1 -> Element/1

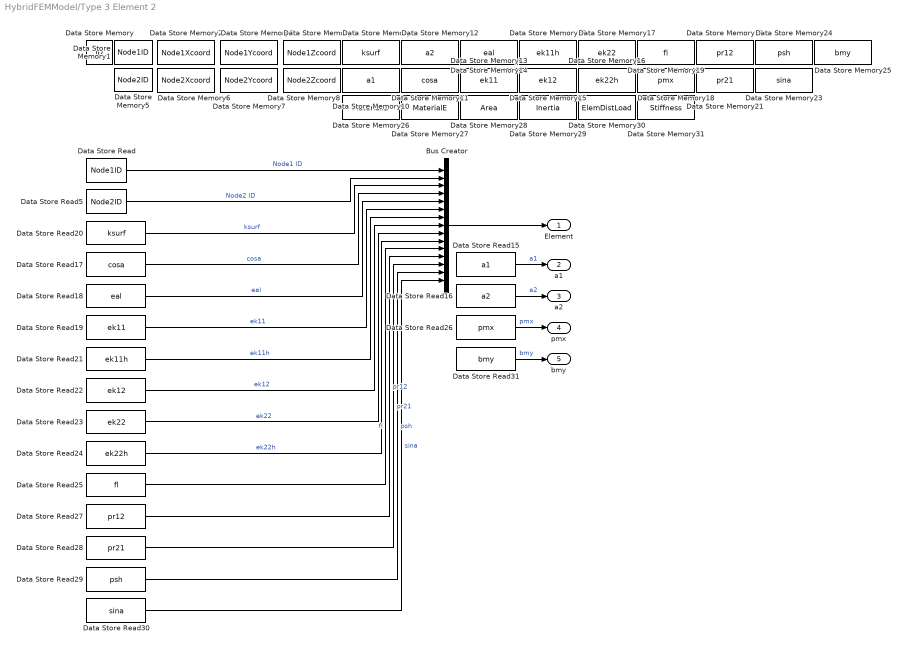
== system HybridFEMModel/Type 3 Element 2 ==
  Bus Creator : BusCreator  Inputs=15
  Data Store Memory : DataStoreMemory  DataStoreName=ID  InitialValue=Elements(id).ID  OutDataType=sfix(16)  OutScaling=2^0
  Data Store Memory1 : DataStoreMemory  DataStoreName=Node1ID  InitialValue=Elements(id).Nodes(1).ID  OutDataType=sfix(16)  OutScaling=2^0
  Data Store Memory10 : DataStoreMemory  DataStoreName=a1  InitialValue=Elements(id).a1  OutDataType=sfix(16)  OutScaling=2^0
  Data Store Memory11 : DataStoreMemory  DataStoreName=cosa  InitialValue=Elements(id).cosa  OutDataType=sfix(16)  OutScaling=2^0
  Data Store Memory12 : DataStoreMemory  DataStoreName=a2  InitialValue=Elements(id).a2  OutDataType=sfix(16)  OutScaling=2^0
  Data Store Memory13 : DataStoreMemory  DataStoreName=ek11  InitialValue=Elements(id).ek11  OutDataType=sfix(16)  OutScaling=2^0
  Data Store Memory14 : DataStoreMemory  DataStoreName=eal  InitialValue=Elements(id).eal  OutDataType=sfix(16)  OutScaling=2^0
  Data Store Memory15 : DataStoreMemory  DataStoreName=ek12  InitialValue=Elements(id).ek12  OutDataType=sfix(16)  OutScaling=2^0
  Data Store Memory16 : DataStoreMemory  DataStoreName=ek22h  InitialValue=Elements(id).ek22h  OutDataType=sfix(16)  OutScaling=2^0
  Data Store Memory17 : DataStoreMemory  DataStoreName=ek22  InitialValue=Elements(id).ek22  OutDataType=sfix(16)  OutScaling=2^0
  Data Store Memory18 : DataStoreMemory  DataStoreName=pmx  InitialValue=Elements(id).pmx  OutDataType=sfix(16)  OutScaling=2^0
  Data Store Memory19 : DataStoreMemory  DataStoreName=fl  InitialValue=Elements(id).fl  OutDataType=sfix(16)  OutScaling=2^0
  Data Store Memory2 : DataStoreMemory  DataStoreName=Node1Xcoord  InitialValue=Elements(id).Nodes(1).Xcoord  OutDataType=sfix(16)  OutScaling=2^0
  Data Store Memory20 : DataStoreMemory  DataStoreName=ek11h  InitialValue=Elements(id).ek11h  OutDataType=sfix(16)  OutScaling=2^0
  Data Store Memory21 : DataStoreMemory  DataStoreName=pr21  InitialValue=Elements(id).pr21  OutDataType=sfix(16)  OutScaling=2^0
  Data Store Memory22 : DataStoreMemory  DataStoreName=pr12  InitialValue=Elements(id).pr12  OutDataType=sfix(16)  OutScaling=2^0
  Data Store Memory23 : DataStoreMemory  DataStoreName=sina  InitialValue=Elements(id).sina  OutDataType=sfix(16)  OutScaling=2^0
  Data Store Memory24 : DataStoreMemory  DataStoreName=psh  InitialValue=Elements(id).psh  OutDataType=sfix(16)  OutScaling=2^0
  Data Store Memory25 : DataStoreMemory  DataStoreName=bmy  InitialValue=Elements(id).bmy  OutDataType=sfix(16)  OutScaling=2^0
  Data Store Memory26 : DataStoreMemory  DataStoreName=MaterialID  InitialValue=Elements(id).Material.ID  OutDataType=sfix(16)  OutScaling=2^0
  Data Store Memory27 : DataStoreMemory  DataStoreName=MaterialE  InitialValue=Elements(id).Material.E  OutDataType=sfix(16)  OutScaling=2^0
  Data Store Memory28 : DataStoreMemory  DataStoreName=Area  InitialValue=Elements(id).Area  OutDataType=sfix(16)  OutScaling=2^0
  Data Store Memory29 : DataStoreMemory  DataStoreName=Inertia  InitialValue=Elements(id).Inertia  OutDataType=sfix(16)  OutScaling=2^0
  Data Store Memory3 : DataStoreMemory  DataStoreName=Node1Ycoord  InitialValue=Elements(id).Nodes(1).Ycoord  OutDataType=sfix(16)  OutScaling=2^0
  Data Store Memory30 : DataStoreMemory  DataStoreName=ElemDistLoad  InitialValue=Elements(id).ElemDistLoad  OutDataType=sfix(16)  OutScaling=2^0
  Data Store Memory31 : DataStoreMemory  DataStoreName=Stiffness  InitialValue=Elements(id).Stiffness  OutDataType=sfix(16)  OutScaling=2^0
  Data Store Memory4 : DataStoreMemory  DataStoreName=Node1Zcoord  InitialValue=Elements(id).Nodes(1).Zcoord  OutDataType=sfix(16)  OutScaling=2^0
  Data Store Memory5 : DataStoreMemory  DataStoreName=Node2ID  InitialValue=Elements(id).Nodes(2).ID  OutDataType=sfix(16)  OutScaling=2^0
  Data Store Memory6 : DataStoreMemory  DataStoreName=Node2Xcoord  InitialValue=Elements(id).Nodes(2).Xcoord  OutDataType=sfix(16)  OutScaling=2^0
  Data Store Memory7 : DataStoreMemory  DataStoreName=Node2Ycoord  InitialValue=Elements(id).Nodes(2).Ycoord  OutDataType=sfix(16)  OutScaling=2^0
  Data Store Memory8 : DataStoreMemory  DataStoreName=Node2Zcoord  InitialValue=Elements(id).Nodes(2).Zcoord  OutDataType=sfix(16)  OutScaling=2^0
  Data Store Memory9 : DataStoreMemory  DataStoreName=ksurf  InitialValue=Elements(id).ksurf  OutDataType=sfix(16)  OutScaling=2^0
  Data Store Read : DataStoreRead  DataStoreName=Node1ID  SampleTime=SampleRate
  Data Store Read15 : DataStoreRead  DataStoreName=a1  SampleTime=SampleRate
  Data Store Read16 : DataStoreRead  DataStoreName=a2  SampleTime=SampleRate
  Data Store Read17 : DataStoreRead  DataStoreName=cosa  SampleTime=SampleRate
  Data Store Read18 : DataStoreRead  DataStoreName=eal  SampleTime=SampleRate
  Data Store Read19 : DataStoreRead  DataStoreName=ek11  SampleTime=SampleRate
  Data Store Read20 : DataStoreRead  DataStoreName=ksurf  SampleTime=SampleRate
  Data Store Read21 : DataStoreRead  DataStoreName=ek11h  SampleTime=SampleRate
  Data Store Read22 : DataStoreRead  DataStoreName=ek12  SampleTime=SampleRate
  Data Store Read23 : DataStoreRead  DataStoreName=ek22  SampleTime=SampleRate
  Data Store Read24 : DataStoreRead  DataStoreName=ek22h  SampleTime=SampleRate
  Data Store Read25 : DataStoreRead  DataStoreName=fl  SampleTime=SampleRate
  Data Store Read26 : DataStoreRead  DataStoreName=pmx  SampleTime=SampleRate
  Data Store Read27 : DataStoreRead  DataStoreName=pr12  SampleTime=SampleRate
  Data Store Read28 : DataStoreRead  DataStoreName=pr21  SampleTime=SampleRate
  Data Store Read29 : DataStoreRead  DataStoreName=psh  SampleTime=SampleRate
  Data Store Read30 : DataStoreRead  DataStoreName=sina  SampleTime=SampleRate
  Data Store Read31 : DataStoreRead  DataStoreName=bmy  SampleTime=SampleRate
  Data Store Read5 : DataStoreRead  DataStoreName=Node2ID  SampleTime=SampleRate
  Element : Outport  OutDataType=sfix(16)  OutScaling=2^0
  a1 : Outport  Port=2  OutDataType=sfix(16)  OutScaling=2^0
  a2 : Outport  Port=3  OutDataType=sfix(16)  OutScaling=2^0
  pmx : Outport  Port=4  OutDataType=sfix(16)  OutScaling=2^0
  bmy : Outport  Port=5  OutDataType=sfix(16)  OutScaling=2^0
  wires:
  Bus Creator/1 -> Element/1
  Data Store Read/1 -> Bus Creator/1  "Node1 ID"
  Data Store Read5/1 -> Bus Creator/2  "Node2 ID"
  Data Store Read20/1 -> Bus Creator/3  "ksurf"
  Data Store Read17/1 -> Bus Creator/4  "cosa"
  Data Store Read18/1 -> Bus Creator/5  "eal"
  Data Store Read19/1 -> Bus Creator/6  "ek11"
  Data Store Read21/1 -> Bus Creator/7  "ek11h"
  Data Store Read22/1 -> Bus Creator/8  "ek12"
  Data Store Read23/1 -> Bus Creator/9  "ek22"
  Data Store Read24/1 -> Bus Creator/10  "ek22h"
  Data Store Read25/1 -> Bus Creator/11  "fl"
  Data Store Read27/1 -> Bus Creator/12  "pr12"
  Data Store Read28/1 -> Bus Creator/13  "pr21"
  Data Store Read29/1 -> Bus Creator/14  "psh"
  Data Store Read30/1 -> Bus Creator/15  "sina"
  Data Store Read15/1 -> a1/1  "a1"
  Data Store Read16/1 -> a2/1  "a2"
  Data Store Read26/1 -> pmx/1  "pmx"
  Data Store Read31/1 -> bmy/1  "bmy"
